simulink model "sistema_P"  (R2026a)
settings: Solver=ode4  StopTime=16.5  FixedStep=1e-3
undefined symbols (not defined in the file or in its folder): C_k
libraries: cstblocks_lti x1, simulink x1
settings Model: Creator=Dante P  LastModifiedBy=Dante P

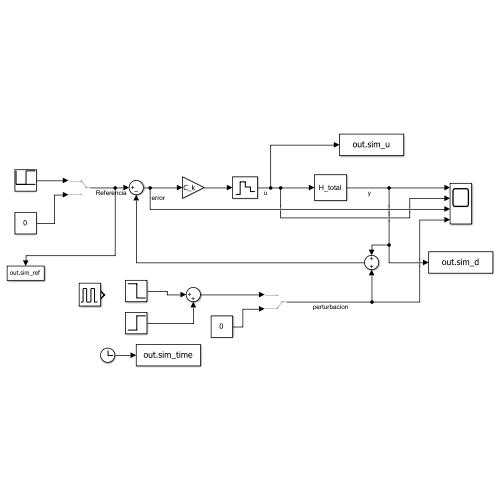
[thumbnail: Simulink's stored preview of the top-level diagram]
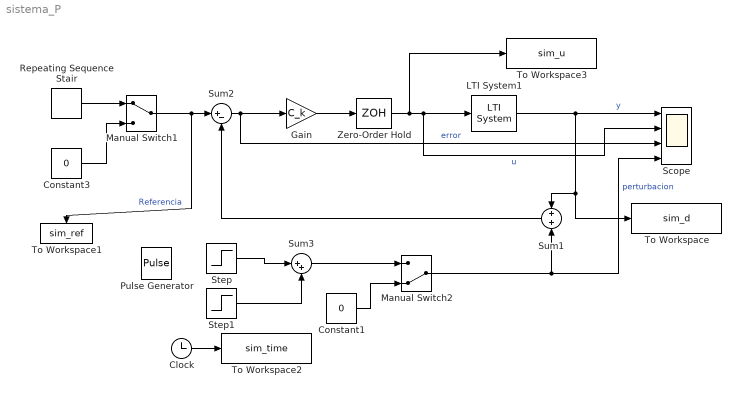
== system sistema_P ==
  Clock : Clock
  Constant1 : Constant  Value=0
  Constant3 : Constant  Value=0
  Gain : Gain  Gain=C_k
  LTI System1 : cstblocks_lti/LTI System  sys=H_total  IC=x0  PadeOrder=0
  Manual Switch1 : ManualSwitch
  Manual Switch2 : ManualSwitch  CurrentSetting=0
  Pulse Generator : DiscretePulseGenerator  PulseType=Time based  Amplitude=5  Period=15  PulseWidth=0.1  PhaseDelay=3
  Repeating Sequence Stair : simulink/Sources/Repeating Sequence Stair  OutValues=[0 10].'  tsamp=10  OutMin=[]  OutMax=[]  OutDataTypeStr=double  OutputDataTypeScalingMode=double  OutDataType=fixdt(0,8)  ConRadixGroup=Best Precision: Vector-wise  OutScaling=2^-12
  Scope : Scope  NumInputPorts=4
      settings: ActiveDisplayYMinimum=-113.20134224248869  ActiveDisplayYMaximum=18.81208018239828
  Step : Step  Time=5  FinalValue=-48  SampleTime=0
  Step1 : Step  Time=5.05  FinalValue=48  SampleTime=0
  Sum1 : Sum  Inputs=+|+
  Sum2 : Sum  Inputs=|+-
  Sum3 : Sum  Inputs=|++
  To Workspace : ToWorkspace  VariableName=sim_d  SampleTime=0.02
  To Workspace1 : ToWorkspace  VariableName=sim_ref  SampleTime=0.02
  To Workspace2 : ToWorkspace  VariableName=sim_time  SampleTime=0.02
  To Workspace3 : ToWorkspace  VariableName=sim_u  SampleTime=0.02
  Zero-Order Hold : ZeroOrderHold  SampleTime=0.02
  wires:
  Sum2/1 -> Gain/1, Scope/3  "error"
  Constant3/1 -> Manual Switch1/2
  Manual Switch1/1 -> To Workspace1/1, Sum2/1  "Referencia"
  Constant1/1 -> Manual Switch2/2
  Manual Switch2/1 -> Scope/4, Sum1/2  "perturbacion"
  Sum1/1 -> Sum2/2
  Repeating Sequence Stair/1 -> Manual Switch1/1
  Clock/1 -> To Workspace2/1
  Gain/1 -> Zero-Order Hold/1
  Zero-Order Hold/1 -> To Workspace3/1, Scope/2, LTI System1/1  "u"
  LTI System1/1 -> Scope/1, To Workspace/1, Sum1/1  "y"
  Step/1 -> Sum3/1
  Step1/1 -> Sum3/2
  Sum3/1 -> Manual Switch2/1
